simulink model "FMBroadcastTransmitterR21b"  (R2021b)
settings: Solver=VariableStepAuto  StartTime=0.0  StopTime=inf  RelTol=1e-3
undefined symbols (not defined in the file): Fs, ip, usb
libraries: dspvision x3, commanabbnd3 x3, plutoradiolib x2, audiosources x2
settings Model: Creator=rohith  LastModifiedBy=csanchis
settings SolverCC: AlgebraicLoopSolver=TrustRegion
settings DebuggingCC: SFMachineParentedDataDiag=warning

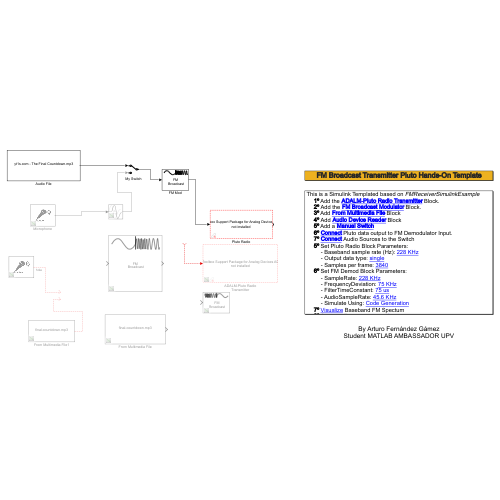
[thumbnail: Simulink's stored preview of the top-level diagram]
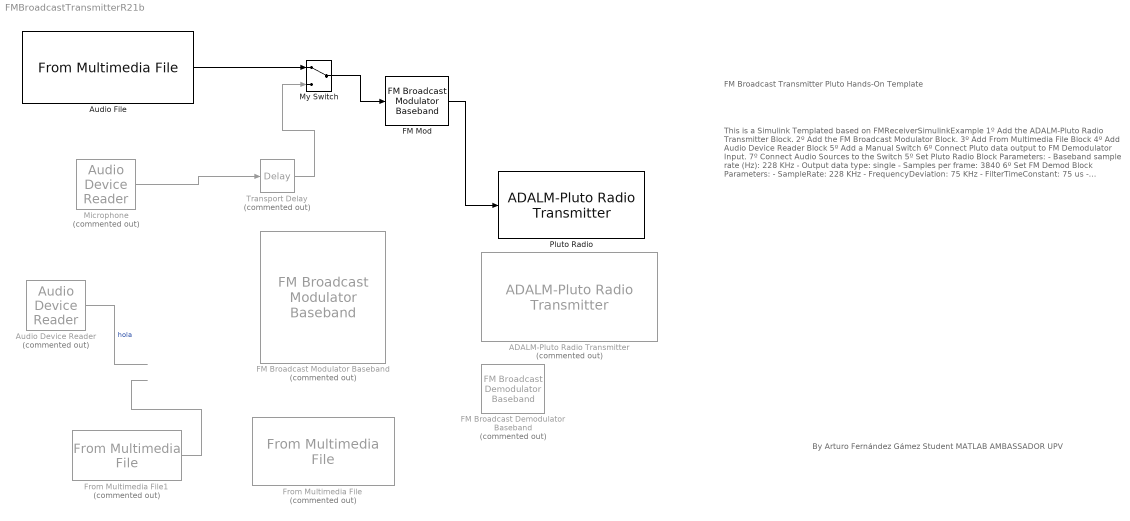
== system FMBroadcastTransmitterR21b ==
  note: By Arturo Fernández Gámez
      | Student MATLAB AMBASSADOR UPV
  note: FM Broadcast Transmitter Pluto Hands-On Template
  note: This is a Simulink Templated based on FMReceiverSimulinkExample
      | 1º Add the ADALM-Pluto Radio Transmitter Block.
      | 2º Add the FM Broadcast Modulator Block.
      | 3º Add From Multimedia File Block
      | 4º Add Audio Device Reader Block
      | 5º Add a Manual Switch
      | 6º Connect Pluto data output to FM Demodulator Input.
      | 7º Connect Audio Sources to the Switch
      | 5º Set Pluto Radio Block Parameters:
      | - Baseband sample rate (Hz): 228 KHz
      | - Output data type: single
      | - Samples per frame: 3840
      | 6º Set FM Demod Block Parameters:
      | - SampleRate: 228 KHz
      | - FrequencyDeviation: 75 KHz
      | - FilterTimeConstant: 75 us
      | - AudioSampleRate: 45.6 KHz
      | - Simulate Using: Code Generation
      | 7º Visualize Baseband FM Spectum
      | 8º Create a Frequency Input Component
  ADALM-Pluto Radio Transmitter : plutoradiolib/ADALM-Pluto Radio Transmitter  Commented=on  RadioID=usb:0  uri=ip:10.0.0.200  CenterFrequencySource=Dialog  CenterFrequency=109e6  GainSource=Dialog  Gain=-1.5  ChannelMapping=1  BasebandSampleRate=1e6  UnderflowOutputPort=off  ShowAdvancedProperties=off  UseCustomFilter=off  filtPathRates=[737280000 11520000 3840000 1920000 960000 240000]  filtCoefficients=[-192 82 85 -215 228 -102 -110 290 -318 145 160 -426 471 -215 -238 633 -697 318 349 -923 1009 -457 -498 1309 -1423 640 693 -1812 1959 -876 -945 2458 -2647 1180 1268 -3290 3534 -1572 -1688 4375 -4698 2091 2247 -5836 6284 -2807 -3031 7918 -8588 3870 4225 -11182 12324 -5662 -6330 17255 -19735 9507 11312 -33568 43355 -25227 -42139 305542 305542 -42139 -25227 43355 -33568 11312 9507 -19735 17255 -6330 -5662 12324 -11182 4225 3870 -8588 7918 -3031 -2807 6284 -5836 2247 2091 -4698 4375 -1688 -1572 3534 -3290 1268 1180 -2647 2458 -945 -876 1959 -1812 693 640 -1423 1309 -498 -457 1009 -923 349 318 -697 633 -238 -215 471 -426 160 145 -318 290 -110 -102 228 -215 85 82 -192]  filtCoefficientSize=128  filtDecimInterpFactor=4  filtGain=-12  filtRFBandwidth=18000000  filterConfigStruct=struct()  DataSourceSelect=Input Port  DDSTone1Freq=5e3  DDSTone2Freq=10e3  DDSTone1Scale=0.5  DDSTone2Scale=0.25  DataTimeout=Inf  FrequencyCorrection=0  ENSMPinControlMode=None  BISTLoopbackMode=Disabled  BISTToneInject=Disabled  BISTSignalGen=PRBS  BISTToneFreq=Fs/32  BISTToneLevel=0
      settings: SourceProductBaseCode=PLUTO
  Audio Device Reader : audiosources/Audio Device Reader  Commented=on  Driver=DirectSound  Device=Default  SampleRate=44100  NumChannels=2  SamplesPerFrame=2000  BitDepth=16-bit integer  NumBuffers=10  DefaultInputChannelMapping=on  InputChannelMapping=1:2  OutputNumOverrunSamples=off  OutputDataType=double  DriverIdx=1  DeviceWarnFlag=''
      settings: SourceProductBaseCode=AU
  Audio File : dspvision/From Multimedia File  inputFilename=C:\Users\Arturo Fernández\Documents\UPV\MATLAB AMBASSADOR\Pluto SDR Workshop\yt1s.com - The Final Countdown.mp3  readRange=[1 Inf]  loop=on  numPlays=inf  outputStreams=Audio only  videoDataType=single  audioDataType=double  inheritSampleTime=on  userDefinedSampleTime=1/30  noAudioOutput=off  isIntensityVideo=off  fourcc=RGB  colorVideoFormat=Separate color signals  outputEOF=off  dataOrg=Column-major  audioFrameSize=2000  computeAudioFrameSize=off  outSamplingMode=Sample based
  FM Broadcast Demodulator Baseband : commanabbnd3/FM Broadcast Demodulator Baseband  Commented=on  SampleRate=240e3  FrequencyDeviation=2000  FilterTimeConstant=75e-6  AudioSampleRate=48000  PlaySound=on  BufferSize=4096  Stereo=off  RBDS=off  RBDSSamplesPerSymbol=10  RBDSCostasLoop=off  SimulateUsing=Code generation
      settings: SourceProductBaseCode=CM
  FM Broadcast Modulator Baseband : commanabbnd3/FM Broadcast Modulator Baseband  Commented=on  SampleRate=240e3  FrequencyDeviation=2000  FilterTimeConstant=75e-6  AudioSampleRate=2000  Stereo=on  RBDS=off  RBDSSamplesPerSymbol=10  SimulateUsing=Code generation
      settings: SourceProductBaseCode=CM
  FM Mod : commanabbnd3/FM Broadcast Modulator Baseband  SampleRate=228e3  FrequencyDeviation=50e3  FilterTimeConstant=50e-6  AudioSampleRate=48e3  Stereo=on  RBDS=off  RBDSSamplesPerSymbol=10  SimulateUsing=Code generation
      settings: SourceProductBaseCode=CM
  From Multimedia File : dspvision/From Multimedia File  Commented=on  inputFilename=C:\Users\Arturo Fernández\Documents\UPV\MATLAB AMBASSADOR\Pluto SDR Workshop\final-countdown.mp3  readRange=[1 Inf]  loop=on  numPlays=inf  outputStreams=Audio only  videoDataType=single  audioDataType=double  inheritSampleTime=on  userDefinedSampleTime=1/30  noAudioOutput=off  isIntensityVideo=off  fourcc=RGB  colorVideoFormat=Separate color signals  outputEOF=off  dataOrg=Column-major  audioFrameSize=2000  computeAudioFrameSize=off  outSamplingMode=Sample based
  From Multimedia File1 : dspvision/From Multimedia File  Commented=on  inputFilename=C:\Users\Arturo Fernández\Documents\UPV\MATLAB AMBASSADOR\Pluto SDR Workshop\final-countdown.mp3  readRange=[1 Inf]  loop=on  numPlays=inf  outputStreams=Audio only  videoDataType=single  audioDataType=double  inheritSampleTime=on  userDefinedSampleTime=1/30  noAudioOutput=off  isIntensityVideo=off  fourcc=RGB  colorVideoFormat=Separate color signals  outputEOF=off  dataOrg=Column-major  audioFrameSize=2000  computeAudioFrameSize=off  outSamplingMode=Sample based
  Microphone : audiosources/Audio Device Reader  Commented=on  Driver=DirectSound  Device=Default  SampleRate=44100  NumChannels=2  SamplesPerFrame=2000  BitDepth=16-bit integer  NumBuffers=10  DefaultInputChannelMapping=on  InputChannelMapping=1:2  OutputNumOverrunSamples=off  OutputDataType=double  DriverIdx=1  DeviceWarnFlag=''
      settings: SourceProductBaseCode=AU
  My Switch : ManualSwitch
  Pluto Radio : plutoradiolib/ADALM-Pluto Radio Transmitter  RadioID=usb:0  uri=ip:10.0.0.200  CenterFrequencySource=Dialog  CenterFrequency=109e6  GainSource=Dialog  Gain=0  ChannelMapping=1  BasebandSampleRate=228e3  UnderflowOutputPort=on  ShowAdvancedProperties=off  UseCustomFilter=off  filtPathRates=[737280000 11520000 3840000 1920000 960000 240000]  filtCoefficients=[-192 82 85 -215 228 -102 -110 290 -318 145 160 -426 471 -215 -238 633 -697 318 349 -923 1009 -457 -498 1309 -1423 640 693 -1812 1959 -876 -945 2458 -2647 1180 1268 -3290 3534 -1572 -1688 4375 -4698 2091 2247 -5836 6284 -2807 -3031 7918 -8588 3870 4225 -11182 12324 -5662 -6330 17255 -19735 9507 11312 -33568 43355 -25227 -42139 305542 305542 -42139 -25227 43355 -33568 11312 9507 -19735 17255 -6330 -5662 12324 -11182 4225 3870 -8588 7918 -3031 -2807 6284 -5836 2247 2091 -4698 4375 -1688 -1572 3534 -3290 1268 1180 -2647 2458 -945 -876 1959 -1812 693 640 -1423 1309 -498 -457 1009 -923 349 318 -697 633 -238 -215 471 -426 160 145 -318 290 -110 -102 228 -215 85 82 -192]  filtCoefficientSize=128  filtDecimInterpFactor=4  filtGain=-12  filtRFBandwidth=18000000  filterConfigStruct=struct()  DataSourceSelect=Input Port  DDSTone1Freq=5e3  DDSTone2Freq=10e3  DDSTone1Scale=0.5  DDSTone2Scale=0.25  DataTimeout=Inf  FrequencyCorrection=0  ENSMPinControlMode=None  BISTLoopbackMode=Disabled  BISTToneInject=Disabled  BISTSignalGen=PRBS  BISTToneFreq=Fs/32  BISTToneLevel=0
      settings: SourceProductBaseCode=PLUTO
  Transport Delay : TransportDelay  Commented=on  DelayTime=5
  wires:
  Audio Device Reader/1 -> ?  "hola"
  Microphone/1 -> Transport Delay/1
  My Switch/1 -> FM Mod/1
  Transport Delay/1 -> My Switch/2
  Audio File/1 -> My Switch/1
  From Multimedia File1/1 -> ?
  FM Mod/1 -> Pluto Radio/1
  ? -> ADALM-Pluto Radio Transmitter/1
